simulink library "Backhoe_Lib"  (R2014a)
settings: Solver=ode45  StartTime=0.0  StopTime=10.0  RelTol=1e-3
undefined symbols (not defined in the file): cylinderGray, gcbh, pistonGray, rhoSteel, simmechanics, X, Y, Z
libraries: sm_lib x40, Backhoe_Lib x7, fl_lib x7, nesl_utility x2
(part 1 of 2)
Description:
  | Copyright 2008-2014 The MathWorks, Inc.
settings Model: Creator=MathWorks  LastModifiedBy=Olli

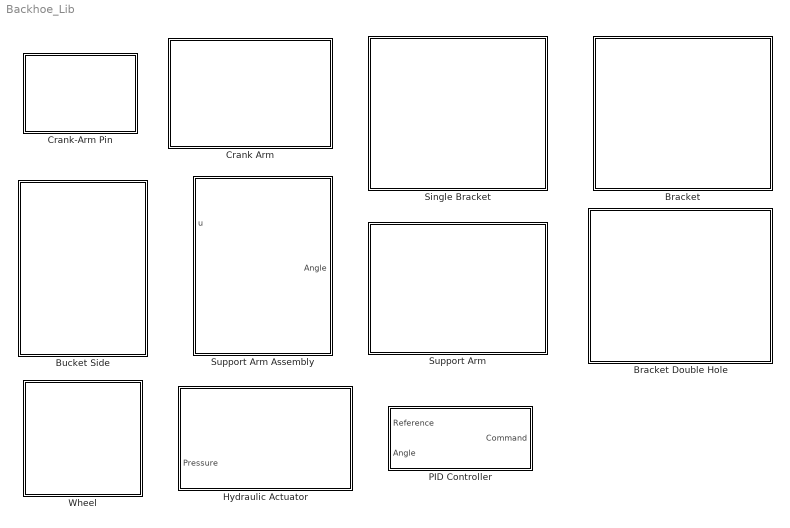
== system Backhoe_Lib ==
  Bracket : Subsystem  mask(Bracket){Hbracket=0.75, Wbracket=0.75, Tbracket=0.15, Dbracket=0.8, Hhole=0.5, Rhole=0.075, circlePoints=25, bracketColor=[0.8 0.8 0], rho=7780}
      mask prompts: Hbracket "Hbracket [m]"; Wbracket "Wbracket [m]"; Tbracket "Tbracket [m]"; Dbracket "Dbracket [m]"; Hhole "Hhole [m]"; Rhole "Rhole [m]"; circlePoints "Circle Mesh Resolution"; bracketColor "Bracket Color"; rho "Density [kg/m^3]"
      mask help:
      | Consists of the backhoe bracket assembly.
      |
      | Attachment points are:
      | B: The base of the bracket.
      | H: The center point between the two holes, which is configured for Revolute joints.
      |
      | Click on Help to view a schematic of the bracket, its configurable dimension parameters and attachment points (in red).
      mask init:
      | bracketPoints = [];
      | 
      | %% Bracket mold.
      | y = Hbracket - (Wbracket/2);
      | for i = 0:circlePoints
      |     angle = (i/circlePoints)*pi;
      |     bracketPoints = [bracketPoints; ...
      |                     (Wbracket/2)*cos(angle) (y+(Wbracket/2)*sin(angle))];
      | end
      | bracketPoints = [bracketPoints; ...
      |                  -Wbracket/2 0;0 0];
      |              
      | %% Hole
      | for i = 0:circlePoints*2
      |     angle = -pi/2 - (i/circlePoints)*pi;
      |     bracketPoints = [bracketPoints; ...
      |                     Rhole*cos(angle) (Hhole+(Rhole*sin(angle)))];
      | end
      | bracketPoints = [bracketPoints; ...
      |                  0 0;Wbracket/2 0];
      |                  
      | %% Uncomment to plot the cross-sections
      | % close all;
      | % figure;
      | % plot(bracketPoints(:,1),bracketPoints(:,2),'b*-');
      mask Help: web('Backhoe_Bracket.html');
      mask Display:
      | image(imread('Backhoe_Bracket_IMAGE.png'));
      | port_label('lconn',1,'B');
      | port_label('rconn',1,'H');
  Bracket Double Hole : Subsystem  mask(Bracket Double Hole){Hbracket=1, Wbracket=2, Tbracket=0.15, Dbracket=0.8, Hhole=0.5, Dhole=1.5, Rhole=0.1, Rfillet=0.4, Nc=25, bracketColor=[0.8 0.8 0], rho=7780}
      mask prompts: Hbracket "Hbracket [m]"; Wbracket "Wbracket [m]"; Tbracket "Tbracket [m]"; Dbracket "Dbracket [m]"; Hhole "Hhole [m]"; Dhole "Dhole [m]"; Rhole "Rhole [m]"; Rfillet "Rfillet [m]"; Nc "Circle Resolution (pts/rev)"; bracketColor "Bracket Color"; rho "Density [kg/m^3]"
      mask help:
      | Consists of the backhoe double-hole bracket assembly.
      |
      | Attachment points are:
      | B: The base of the bracket.
      | HL: The center point between the two left holes, which is configured for Revolute joints.
      | HR: The center point between the two right holes, which is configured for Revolute joints.
      |
      | Click on Help to view a schematic of the bracket, its configurable dimension parameters and attachment points (in red).
      mask init:
      | %% Right Hole
      | bracketPoints = [0 0; Dhole/2 0];
      | angle = linspace(-pi/2,-5*pi/2,Nc)';
      | bracketPoints = [bracketPoints; ...
      |                  (Dhole/2+Rhole*cos(angle)) (Hhole+Rhole*sin(angle))];
      | bracketPoints = [bracketPoints; Dhole/2 0];                 
      | 
      | %% Bracket Outer Boundary
      | bracketPoints = [bracketPoints; Wbracket/2 0];
      | x = Wbracket/2 - Rfillet;
      | y = Hbracket - Rfillet;
      | angle = linspace(0,pi/2,Nc/4)';
      | bracketPoints = [bracketPoints; ...
      |                  (x+Rfillet*cos(angle)) (y+Rfillet*sin(angle))];
      | 
      | angle = linspace(pi/2,pi,Nc/4)';             
      | bracketPoints = [bracketPoints; ...
      |                  (-x+Rfillet*cos(angle)) (y+Rfillet*sin(angle))];
      | bracketPoints = [bracketPoints; -Wbracket/2 0];
      |                  
      | %% Left Hole
      | bracketPoints = [bracketPoints;-Dhole/2 0];
      | angle = linspace(-pi/2,-5*pi/2,Nc)';
      | bracketPoints = [bracketPoints; ...
      |                  (-Dhole/2+Rhole*cos(angle)) (Hhole+Rhole*sin(angle))];
      | bracketPoints = [bracketPoints;-Dhole/2 0];
      mask Help: web('Backhoe_Bracket2.html');
      mask Display:
      | image(imread('Backhoe_Bracket2_IMAGE.png'));
      | port_label('lconn',1,'B');
      | port_label('rconn',1,'HR');
      | port_label('rconn',2,'HL');
  Bucket Side : Subsystem  mask(Bucket Side){bucketUpper=1.3, bucketLower=2, bucketHeight=2, bucketThickness=0.05, chordAngle=pi/6, Nc=45, color=[0.8 0.8 0], rho=7780}
      mask prompts: bucketUpper "Wupper [m]"; bucketLower "Wlower [m]"; bucketHeight "Hbucket [m]"; bucketThickness "Tbucket [m]"; chordAngle "alpha [radians]"; Nc "Circle Resolution (pts/rev)"; rho "Density [kg/m^3]"
      mask help:
      | Consists of the backhoe bucket side plate, which is used as an auxiliary library block inside the Bucket block.
      |
      | Click on Help to view a schematic of the bucket, its configurable dimension parameters and attachment points (in red).
      mask init:
      | bucketRadius = bucketHeight/(2*cos(chordAngle));
      | 
      | Nch = Nc*(pi-2*chordAngle)/(2*pi);
      | angle = linspace(-pi/2+chordAngle, pi/2-chordAngle,Nch)'; 
      | bucketSide = [(bucketRadius*cos(angle)-bucketRadius*sin(chordAngle)) ...
      |        bucketRadius*sin(angle)];
      | 
      | bucketSide = [ bucketSide; ...
      |               -bucketUpper bucketHeight/2; ...
      |               -bucketLower -(bucketHeight/2 - bucketThickness);...
      |               -bucketLower -bucketHeight/2];
      mask Help: web('Backhoe_Bucket.html');
      mask Display:
      | image(imread('Backhoe_Bucketside_IMAGE.png'));
      | port_label('rconn',1,'B');
  Crank Arm : Subsystem  mask(Crank Arm){L=1, W=0.25, T=0.1, D=0.75, R=0.05, Nc=25, color=[0.8 0.8 0], rho=7780}
      mask prompts: L "L [m]"; W "W [m]"; T "T [m]"; D "D [m]"; R "Rhole [m]"; Nc "Circle Resolution (pts/rev)"; rho "Density [kg/m^3]"
      mask help:
      | Parameterized bar with rounded ends and two holes for attachment.
      |
      | Attachment points are the left (L) and right (R) holes of the crank arm, which are configured for Revolute Joints.
      |
      | Click on Help to view a schematic of the bracket, its configurable dimension parameters and attachment points (in red).
      mask init:
      | crankPoints = [];
      | 
      | % Crank 1
      | x = (L - W)/2;
      | angle = linspace(-pi/2,pi/2,Nc/2)';
      | crankPoints = [crankPoints; ...
      |       (x + W*cos(angle)/2) W*sin(angle)/2];
      |   
      | x = D/2;
      | angle = linspace(pi/2,-3*pi/2,Nc)';
      | crankPoints = [crankPoints; ...
      |       (x + R*cos(angle)) R*sin(angle)];
      | 
      | crankPoints = [crankPoints;x W/2];
      | x = -D/2;
      | crankPoints = [crankPoints;x W/2];
      | 
      | angle = linspace(pi/2,-3*pi/2,Nc)';
      | crankPoints = [crankPoints; ...
      |       (x + R*cos(angle)) R*sin(angle)];
      | 
      | x = -(L - W)/2;
      | angle = linspace(pi/2,3*pi/2,Nc/2)';
      | crankPoints = [crankPoints; ...
      |       (x + W*cos(angle)/2) W*sin(angle)/2];
      mask Help: web('Backhoe_Crankarm.html');
      mask Display:
      | image(imread('Backhoe_Crankarm_IMAGE.png'));
      | port_label('lconn',1,'L');
      | port_label('rconn',1,'R');
  Crank-Arm Pin : Subsystem  mask(Crank Pin){R=0.1, L=1, T=0.1, color=[0.3 0.3 0.3], rho=7780}
      mask prompts: R "Radius [m]"; L "Length [m]"; T "Crank Arm Thickness [m]"; rho "Density [kg/m^3]"
      mask help:
      | Parameterized block for the two pins that extrude from the Upper Arm. These pins connect to the crank arms, which create a four-bar linkage with the Upper Arm and the Bucket.
      |
      | Attachment points are:
      | B: Base of the pin.
      | C: Crank arm attachment point which is configured for Revolute joints.
      mask Display:
      | image(repmat(imread('Backhoe_Crankpin_IMAGE.png'),[1 1 3]));
      | port_label('lconn',1,'C');
      | port_label('rconn',1,'B');
  Hydraulic Actuator : Subsystem  mask(Hydraulic Actuator){Lcyl=2.5, Rcyl=0.2, Lpist=2.5, Rpist=0.1, Lbase=0.65, Wbase=0.35, Rbp=0.075, Lbp=0.8, Whead=0.35, Lhead=0.65, Rhp=0.075, Lhp=0.9, circlePoints=25, cylColor=[0.6 0.6 0.6], rhoCyl=7780, pistColor=[0.4 0.4 0.4], rhoPist=7780, connColor=[0.3 0.3 0.3], rhoConn=7780}
      mask prompts: Lcyl "Lcyl [m]"; Rcyl "Rcyl [m]"; Lpist "Lpist [m]"; Rpist "Rpist [m]"; Lbase "Lbase [m]"; Wbase "Wbase [m]"; Rbp "Rbp [m]"; Lbp "Lbp [m]"; Whead "Whead [m]"; Lhead "Lhead [m]"; Rhp "Rhp [m]"; Lhp "Lhp [m]"; circlePoints "Circle Mesh Resolution"; cylColor "Cylinder Color"; rhoCyl "Cylinder Density [kg/m^3]"; pistColor "Piston Color"; rhoPist "Piston Density [kg/m^3]"; connColor "Connector Color"; rhoConn "Connector Density [kg/m^3]"
      mask help:
      | Consists of the backhoe hydraulic actuator assembly.
      |
      | Zero piston displacement corresponds to the piston and cylinder centers of mass in the same position. Positive piston displacement is outward motion, and negative piston displacement is inward motion.
      |
      | Attachment points are:
      | C: Center of the Cylinder base bracket hole.
      | H: Center of the Piston Head bracket hole.
      | Both attachment points are configured for Revolute joints.
      |
      | The Simulink Signal input port supplies a Pressure value P (in Pa) to a Simscape hydraulic network.
      |
      | Click on Help to view a schematic of the hydraulic actuator, its configurable dimension parameters and attachment points (in red).
      mask init:
      | % Hollow Cylinder cross-section
      | cylSection = [];
      | 
      | for i = 0:2*circlePoints
      |     angle = (i/circlePoints)*pi;
      |     cylSection = [cylSection; Rcyl*cos(angle) Rcyl*sin(angle)];
      | end
      | 
      | for i = 0:2*circlePoints
      |     angle = -(i/circlePoints)*pi;
      |     cylSection = [cylSection; Rpist*cos(angle) Rpist*sin(angle)];
      | end
      mask Help: web('Backhoe_Actuator.html');
      mask Display:
      | image(repmat(imread('Backhoe_Actuator_IMAGE.png'),[1 1 3]));
      | port_label('rconn',1,'H');
      | port_label('lconn',1,'C');
      | port_label('input',1,'P');
  PID Controller : Subsystem  mask(PID Controller){upperLim=inf, lowerLim=-inf, Kp=0, Ki=0, Kd=0, N=0}
      mask prompts: upperLim "Upper Limit [deg]"; lowerLim "Lower Limit [deg]"
      mask help: This block takes in a reference angle and measured angle, and uses a PID Controller with saturation to give a control command.
  Single Bracket : Subsystem  mask(Single Bracket){Hbracket=0.75, Wbracket=0.75, Tbracket=0.15, Hhole=0.5, Rhole=0.075, Nc=25, bracketColor=[0.8 0.8 0], rho=7780}
      mask prompts: Hbracket "Hbracket [m]"; Wbracket "Wbracket [m]"; Tbracket "Tbracket [m]"; Hhole "Hhole [m]"; Rhole "Rhole [m]"; Nc "Circle Resolution (pts/rev)"; bracketColor "Bracket Color"; rho "Density [kg/m^3]"
      mask help:
      | Consists of the backhoe single bracket assembly.
      |
      | Attachment points are:
      | B: The base of the bracket.
      | H: The center point of the hole, which is configured for Revolute joints.
      |
      | Click on Help to view a schematic of the bracket, its configurable dimension parameters and attachment points (in red).
      mask init:
      | bracketPoints = [];
      | 
      | %% Bracket mold.
      | y = Hbracket - (Wbracket/2);
      | angle = linspace(0,pi,Nc/2)';
      | bracketPoints = [(Wbracket/2)*cos(angle) (y+(Wbracket/2)*sin(angle))];
      | bracketPoints = [bracketPoints; ...
      |                  -Wbracket/2 0;0 0];
      |              
      | %% Hole
      | angle = linspace(3*pi/2,-pi/2,Nc)';
      | bracketPoints = [bracketPoints; ...
      |                  Rhole*cos(angle) (Hhole+(Rhole*sin(angle)))];
      | bracketPoints = [bracketPoints; ...
      |                  0 0;Wbracket/2 0];
      mask Help: web('Backhoe_Singlebracket.html');
      mask Display:
      | image(imread('Backhoe_Bracket1_IMAGE.png'));
      | port_label('lconn',1,'B');
      | port_label('rconn',1,'H');
  Support Arm : Subsystem  mask(Support Arm){Larm=2.5, Warm=0.5, Tarm=0.35, Dhole=2, Rhole=0.075, initAngle=45, Lfoot=2, Wfoot=1, Tfoot=0.2, Dconn=1, Hhole=0.3, Rfillet=0.4, Lpin=0.8, circlePoints=25, armColor=[0.8 0.8 0], bracketColor=[0.8 0.65 0], footColor=[0.8 0.8 0], pinColor=[0.3 0.3 0.3], rho=7780}
      mask prompts: Larm "Larm [m]"; Warm "Warm [m]"; Tarm "Tarm [m]"; Dhole "Dhole [m]"; Rhole "Rhole [m]"; initAngle "Initial Arm-Foot Angle [deg]"; Lfoot "Lfoot [m]"; Wfoot "Wfoot [m]"; Tfoot "Tfoot [m]"; Dconn "Dconn [m]"; Hhole "Hhole [m]"; Rfillet "Rfillet [m]"; Lpin "Lpin [m]"; circlePoints "Circle Mesh Resolution"; armColor "Arm Color"; bracketColor "Bracket Color"; footColor "Foot Color"; pinColor "Pin Color"; rho "Density [kg/m^3]"
      mask help:
      | Consists of the backhoe support arm that connects an arm, a bracket and a foot.
      |
      | Attachment points are:
      | SB: The free hole of the crank arm, which connects to the Shoulder Bracket.
      | PH: The free pin of the foot bracket, which connect to the piston head of a hydraulic actuator.
      | Both attachment points are configured for Revolute Joints.
      |
      | Click on Help to view a schematic of the support arm, its configurable dimension parameters and attachment points (in red).
      mask init:
      | armPoints = [];
      | x = (Larm - Warm)/2;
      | for i=0:circlePoints
      |    angle = -pi/2 + (i/circlePoints)*pi;
      |    armPoints = [armPoints; ...
      |       (x + Warm*cos(angle)/2) Warm*sin(angle)/2];
      | end
      | x = Dhole/2;
      | for i=0:circlePoints*2
      |    angle = pi/2 - (i/circlePoints)*pi;
      |    armPoints = [armPoints; ...
      |       (x + Rhole*cos(angle)) Rhole*sin(angle)];   
      | end
      | armPoints = [armPoints;x Warm/2];
      | x = -Dhole/2;
      | armPoints = [armPoints;x Warm/2];
      | for i=0:circlePoints*2
      |    angle = pi/2 - (i/circlePoints)*pi;
      |    armPoints = [armPoints; ...
      |       (x + Rhole*cos(angle)) Rhole*sin(angle)];   
      | end
      | x = -(Larm - Warm)/2;
      | for i=0:circlePoints
      |    angle = pi/2 + (i/circlePoints)*pi;
      |    armPoints = [armPoints; ...
      |       (x + Warm*cos(angle)/2) Warm*sin(angle)/2];
      | end
      mask Help: web('Backhoe_Supportarm.html');
      mask Display:
      | image(imread('Backhoe_Supportarm_IMAGE.png'));
      | port_label('lconn',1,'PH');
      | port_label('rconn',1,'SB');
  Support Arm Assembly : Subsystem  mask(Support Arm Assembly){Hbracket=0.8, Wbracket=1.75, Tbracket=0.15, Dbracket=0.8, HShoulderHole=0.5, DShoulderHole=1, RShoulderHole=0.075, RShoulderFillet=0.4, Larm=2.5, Warm=0.5, Tarm=0.35, Dhole=2, Rhole=0.075, AFAngle=45, Lpin=0.85, Lfoot=2, Wfoot=1, Tfoot=0.2, Dconn=1, Hhole=0.3, Rfillet=0.4, circlePoints=25, shoulderColor=[1 0.6 0], armColor=[1 0.8 0], bracketColor=[1 0.6 0], footColor=[1 0.8 0], pinColor=[0.5 0.5 0.5], pistonGray=pistonGray, cylinderGray=cylinderGray, rho=rhoSteel}
      mask prompts: Hbracket "Hbracket [m]"; Wbracket "Wbracket [m]"; Tbracket "Tbracket [m]"; Dbracket "Dbracket [m]"; HShoulderHole "HShoulderHole [m]"; DShoulderHole "DShoulderHole [m]"; RShoulderHole "RShoulderHole [m]"; RShoulderFillet "RShoulderFillet [m]"; Larm "Larm [m]"; Warm "Warm [m]"; Tarm "Tarm [m]"; Dhole "Dhole [m]"; Rhole "Rhole [m]"; AFAngle "Arm-Foot Angle [deg]"; Lpin "Lpin [m]"; Lfoot "Lfoot [m]"; Wfoot "Wfoot [m]"; Tfoot "Tfoot [m]"; Dconn "Dconn [m]"; Hhole "Hhole [m]"; Rfillet "Rfillet [m]"; circlePoints "Circle Mesh Resolution"; shoulderColor "Shoulder Bracket Color"; armColor "Arm Color"; bracketColor "Foot Bracket Color"; footColor "Foot Color"; pinColor "Pin Color"; pistonGray "Piston Color"; cylinderGray "Cylinder Color"; rho "Density [kg/m^3]"
      mask help:
      | Consists of a backhoe support arm, a shoulder bracket and a hydraulic actuator.
      |
      | Attachment points are:
      | MB: The base of the shoulder bracket, which connects rigidly to the Mounting Base.
      |
      | Inputs and outputs are:
      | u: The pressure to the hydraulic actuator.
      | a: The angle of the support arm, for sensing.
      |
      | Click on Help to view a schematic of the support arm assembly, its configurable dimension parameters and attachment points (in red).
      mask Help: web('Backhoe_Supportassembly.html');
      mask Display:
      | image(imread('Backhoe_Supportassembly_IMAGE.png'));
      | port_label('input',1,'u');
      | port_label('output',1,'a');
      | port_label('lconn',1,'MB');
  Wheel : Subsystem  mask(Wheel){Rwheel=0.5, Rtire=1, Raxle=0.075, W=0.75, circlePoints=30, tireColor=[0.1 0.1 0.1], rhoTire=1500, wheelColor=[0.6 0.6 0.6], rhoWheel=7780}
      mask prompts: Rwheel "Rwheel [m]"; Rtire "Rtire [m]"; Raxle "Raxle [m]"; W "Width [m]"; circlePoints "Circle Point Resolution"; tireColor "Tire Color"; rhoTire "Tire Density [kg/m^3]"; wheelColor "Wheel Color"; rhoWheel "Wheel Density [kg/m^3]"
      mask help:
      | Consists of the backhoe wheel assembly.
      |
      | Attachment points are:
      | A: The center of the wheel's axle.
      mask init:
      | % Wheel
      | wheelPoints = [];
      | for i = 0:circlePoints
      |    angle = pi*i/circlePoints;
      |    wheelPoints = [wheelPoints ; ...
      |                   Rwheel*cos(angle) Rwheel*sin(angle)];
      | end
      | for i = 0:2*circlePoints
      |    angle = pi - pi*i/circlePoints;
      |    wheelPoints = [wheelPoints ; ...
      |                   Raxle*cos(angle) Raxle*sin(angle)];
      | end
      | for i = 0:circlePoints
      |    angle = pi + pi*i/circlePoints;
      |    wheelPoints = [wheelPoints ; ...
      |                   Rwheel*cos(angle) Rwheel*sin(angle)];
      | end
      | 
      | % Tire
      | tirePoints = [];
      | for i = 0:circlePoints
      |    angle = pi*i/circlePoints;
      |    tirePoints = [tirePoints ; ...
      |                   Rtire*cos(angle) Rtire*sin(angle)];
      | end
      | for i = 0:2*circlePoints
      |    angle = pi - pi*i/circlePoints;
      |    tirePoints = [tirePoints ; ...
      |                   Rwheel*cos(angle) Rwheel*sin(angle)];
      | end
      | for i = 0:circlePoints
      |    angle = pi + pi*i/circlePoints;
      |    tirePoints = [tirePoints ; ...
      |                   Rtire*cos(angle) Rtire*sin(angle)];
      | end
      | 
      | % Rim
      | H = W*0.15;
      | k = H/(Rwheel^2);
      | vec = linspace(Rwheel,Raxle,10)';
      | rimPoints = [Raxle 0; vec  H-k*vec.^2];
      mask Display:
      | image(repmat(imread('Backhoe_Wheel_IMAGE.png'),[1 1 3]));
      | port_label('lconn',1,'A');

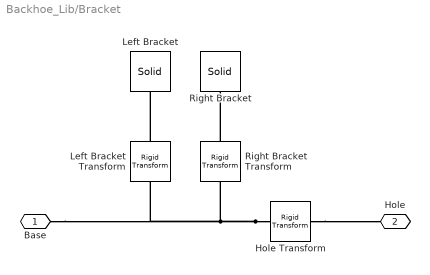
== system Backhoe_Lib/Bracket ==
  Hole Transform : sm_lib/Frames and Transforms/Rigid Transform  TranslationMethod=StandardAxis  TranslationLengthUnit=m  TranslationStandardAxis=+Z  TranslationStandardOffset=Hhole  TranslationCartesianOffset=[0 (Dbracket-Tbracket)/2 Hbracket/2]  TranslationROffset=0  TranslationROffsetUnits=m  TranslationZOffset=0  TranslationZOffsetUnits=m  TranslationThetaOffset=0  TranslationThetaOffsetUnits=deg  RotationMethod=AlignedAxes  RotationAngleUnits=deg  RotationStandardAxis=+X  RotationAngle=90  RotationArbitraryAxis=[0 0 1]  FollAlignAxisA=+X  BaseAlignAxisA=+X  FollAlignAxisB=+Y  BaseAlignAxisB=+Z  BlockFunction=simmechanics.library.frames_transforms.rigid_transform
  Left Bracket : sm_lib/Body Elements/Solid  InertiaType=CalculateFromGeometry  Mass=1  MassUnits=kg  CenterOfMass=[0 0 0]  CenterOfMassUnits=m  MomentsOfInertia=[1 1 1]  MomentsOfInertiaUnits=kg*m^2  ProductsOfInertia=[0 0 0]  ProductsOfInertiaUnits=kg*m^2  DensityBased=on  Density=rho  DensityUnits=kg/(m^3)  GraphicType=FromGeometry  MarkerShape=Sphere  MarkerSize=10  MarkerSizeUnits=m  GraphicVisPropType=SimpleVisualProperties  GraphicDiffuseColor=bracketColor  GraphicSpecularColor=[0.5 0.5 0.5 1.0]  GraphicAmbientColor=[0.15 0.15 0.15 1.0]  GraphicEmissiveColor=[0.0 0.0 0.0 1.0]  GraphicShininess=75  GraphicOpacity=1.0  GeometryShape=GeneralExtrusion  RectangleSize=[1 1]  RectangleSizeUnits=m  BrickDimensions=[Wbracket Tbracket Hbracket ]  BrickDimensionUnits=m  CylinderRadius=1  CylinderRadiusUnits=m  CylinderLength=1  CylinderLengthUnits=m  SphereRadius=1  SphereRadiusUnits=m  EllipsoidRadii=[1 1 1]  EllipsoidRadiiUnits=m  ExtrusionCrossSection=bracketPoints  ExtrusionCrossSectionUnits=m  ExtrusionLength=Tbracket  ExtrusionLengthUnits=m  PolygonNumSides=3  PolygonOuterRadius=1  PolygonOuterRadiusUnits=m  ExtGeomFileUnits=m  RevolutionCrossSection=[1 1; 1 -1; 2 -1; 2 1]  RevolutionCrossSectionUnits=m  RevolutionExtent=Full  RevolutionAngle=180  RevolutionAngleUnits=deg  BlockFunction=simmechanics.library.body_elements.solid
  Left Bracket Transform : sm_lib/Frames and Transforms/Rigid Transform  TranslationMethod=StandardAxis  TranslationLengthUnit=m  TranslationStandardAxis=-Y  TranslationStandardOffset=(Dbracket-Tbracket)/2  TranslationCartesianOffset=[0 0 0]  TranslationROffset=0  TranslationROffsetUnits=m  TranslationZOffset=0  TranslationZOffsetUnits=m  TranslationThetaOffset=0  TranslationThetaOffsetUnits=deg  RotationMethod=AlignedAxes  RotationAngleUnits=deg  RotationStandardAxis=+X  RotationAngle=90  RotationArbitraryAxis=[0 0 1]  FollAlignAxisA=+X  BaseAlignAxisA=+X  FollAlignAxisB=+Y  BaseAlignAxisB=+Z  BlockFunction=simmechanics.library.frames_transforms.rigid_transform
  Right Bracket : sm_lib/Body Elements/Solid  InertiaType=CalculateFromGeometry  Mass=1  MassUnits=kg  CenterOfMass=[0 0 0]  CenterOfMassUnits=m  MomentsOfInertia=[1 1 1]  MomentsOfInertiaUnits=kg*m^2  ProductsOfInertia=[0 0 0]  ProductsOfInertiaUnits=kg*m^2  DensityBased=on  Density=rho  DensityUnits=kg/(m^3)  GraphicType=FromGeometry  MarkerShape=Sphere  MarkerSize=10  MarkerSizeUnits=m  GraphicVisPropType=SimpleVisualProperties  GraphicDiffuseColor=bracketColor  GraphicSpecularColor=[0.5 0.5 0.5 1.0]  GraphicAmbientColor=[0.15 0.15 0.15 1.0]  GraphicEmissiveColor=[0.0 0.0 0.0 1.0]  GraphicShininess=75  GraphicOpacity=1.0  GeometryShape=GeneralExtrusion  RectangleSize=[1 1]  RectangleSizeUnits=m  BrickDimensions=[Wbracket Tbracket Hbracket ]  BrickDimensionUnits=m  CylinderRadius=1  CylinderRadiusUnits=m  CylinderLength=1  CylinderLengthUnits=m  SphereRadius=1  SphereRadiusUnits=m  EllipsoidRadii=[1 1 1]  EllipsoidRadiiUnits=m  ExtrusionCrossSection=bracketPoints  ExtrusionCrossSectionUnits=m  ExtrusionLength=Tbracket  ExtrusionLengthUnits=m  PolygonNumSides=3  PolygonOuterRadius=1  PolygonOuterRadiusUnits=m  ExtGeomFileUnits=m  RevolutionCrossSection=[1 1; 1 -1; 2 -1; 2 1]  RevolutionCrossSectionUnits=m  RevolutionExtent=Full  RevolutionAngle=180  RevolutionAngleUnits=deg  BlockFunction=simmechanics.library.body_elements.solid
  Right Bracket Transform : sm_lib/Frames and Transforms/Rigid Transform  TranslationMethod=StandardAxis  TranslationLengthUnit=m  TranslationStandardAxis=+Y  TranslationStandardOffset=(Dbracket-Tbracket)/2  TranslationCartesianOffset=[0 (Dbracket-Tbracket)/2 Hbracket/2]  TranslationROffset=0  TranslationROffsetUnits=m  TranslationZOffset=0  TranslationZOffsetUnits=m  TranslationThetaOffset=0  TranslationThetaOffsetUnits=deg  RotationMethod=AlignedAxes  RotationAngleUnits=deg  RotationStandardAxis=+X  RotationAngle=90  RotationArbitraryAxis=[0 0 1]  FollAlignAxisA=+X  BaseAlignAxisA=+X  FollAlignAxisB=+Y  BaseAlignAxisB=+Z  BlockFunction=simmechanics.library.frames_transforms.rigid_transform
  Base : PMIOPort  Port=1  Side=Left
  Hole : PMIOPort  Port=2  Side=Right
  connections:
  Hole Transform/LConn1 -- Base/RConn1 -- Left Bracket Transform/LConn1 -- Right Bracket Transform/LConn1
  Right Bracket Transform/RConn1 -- Right Bracket/RConn1
  Left Bracket Transform/RConn1 -- Left Bracket/RConn1
  Hole Transform/RConn1 -- Hole/RConn1

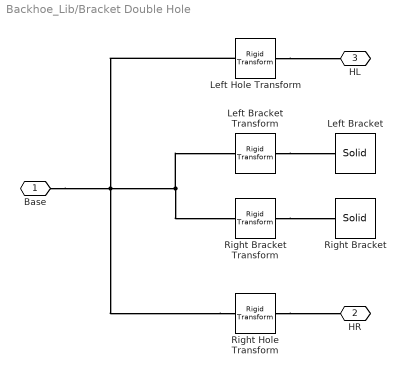
== system Backhoe_Lib/Bracket Double Hole ==
  Left Bracket : sm_lib/Body Elements/Solid  InertiaType=CalculateFromGeometry  Mass=1  MassUnits=kg  CenterOfMass=[0 0 0]  CenterOfMassUnits=m  MomentsOfInertia=[1 1 1]  MomentsOfInertiaUnits=kg*m^2  ProductsOfInertia=[0 0 0]  ProductsOfInertiaUnits=kg*m^2  DensityBased=on  Density=rho  DensityUnits=kg/(m^3)  GraphicType=FromGeometry  MarkerShape=Sphere  MarkerSize=10  MarkerSizeUnits=m  GraphicVisPropType=SimpleVisualProperties  GraphicDiffuseColor=bracketColor  GraphicSpecularColor=[0.5 0.5 0.5 1.0]  GraphicAmbientColor=[0.15 0.15 0.15 1.0]  GraphicEmissiveColor=[0.0 0.0 0.0 1.0]  GraphicShininess=75  GraphicOpacity=1.0  GeometryShape=GeneralExtrusion  RectangleSize=[1 1]  RectangleSizeUnits=m  BrickDimensions=[Wbracket Tbracket Hbracket ]  BrickDimensionUnits=m  CylinderRadius=1  CylinderRadiusUnits=m  CylinderLength=1  CylinderLengthUnits=m  SphereRadius=1  SphereRadiusUnits=m  EllipsoidRadii=[1 1 1]  EllipsoidRadiiUnits=m  ExtrusionCrossSection=bracketPoints  ExtrusionCrossSectionUnits=m  ExtrusionLength=Tbracket  ExtrusionLengthUnits=m  PolygonNumSides=3  PolygonOuterRadius=1  PolygonOuterRadiusUnits=m  ExtGeomFileUnits=m  RevolutionCrossSection=[1 1; 1 -1; 2 -1; 2 1]  RevolutionCrossSectionUnits=m  RevolutionExtent=Full  RevolutionAngle=180  RevolutionAngleUnits=deg  BlockFunction=simmechanics.library.body_elements.solid
  Left Bracket Transform : sm_lib/Frames and Transforms/Rigid Transform  TranslationMethod=StandardAxis  TranslationLengthUnit=m  TranslationStandardAxis=-Y  TranslationStandardOffset=(Dbracket-Tbracket)/2  TranslationCartesianOffset=[0 0 0]  TranslationROffset=0  TranslationROffsetUnits=m  TranslationZOffset=0  TranslationZOffsetUnits=m  TranslationThetaOffset=0  TranslationThetaOffsetUnits=deg  RotationMethod=AlignedAxes  RotationAngleUnits=deg  RotationStandardAxis=+X  RotationAngle=90  RotationArbitraryAxis=[0 0 1]  FollAlignAxisA=+X  BaseAlignAxisA=+X  FollAlignAxisB=+Y  BaseAlignAxisB=+Z  BlockFunction=simmechanics.library.frames_transforms.rigid_transform
  Left Hole Transform : sm_lib/Frames and Transforms/Rigid Transform  TranslationMethod=Cartesian  TranslationLengthUnit=m  TranslationStandardAxis=+Z  TranslationStandardOffset=0  TranslationCartesianOffset=[-Dhole/2 0 Hhole]  TranslationROffset=0  TranslationROffsetUnits=m  TranslationZOffset=0  TranslationZOffsetUnits=m  TranslationThetaOffset=0  TranslationThetaOffsetUnits=deg  RotationMethod=AlignedAxes  RotationAngleUnits=deg  RotationStandardAxis=+Z  RotationAngle=0  RotationArbitraryAxis=[0 0 1]  FollAlignAxisA=+X  BaseAlignAxisA=+X  FollAlignAxisB=+Y  BaseAlignAxisB=+Z  BlockFunction=simmechanics.library.frames_transforms.rigid_transform
  Right Bracket : sm_lib/Body Elements/Solid  InertiaType=CalculateFromGeometry  Mass=1  MassUnits=kg  CenterOfMass=[0 0 0]  CenterOfMassUnits=m  MomentsOfInertia=[1 1 1]  MomentsOfInertiaUnits=kg*m^2  ProductsOfInertia=[0 0 0]  ProductsOfInertiaUnits=kg*m^2  DensityBased=on  Density=rho  DensityUnits=kg/(m^3)  GraphicType=FromGeometry  MarkerShape=Sphere  MarkerSize=10  MarkerSizeUnits=m  GraphicVisPropType=SimpleVisualProperties  GraphicDiffuseColor=bracketColor  GraphicSpecularColor=[0.5 0.5 0.5 1.0]  GraphicAmbientColor=[0.15 0.15 0.15 1.0]  GraphicEmissiveColor=[0.0 0.0 0.0 1.0]  GraphicShininess=75  GraphicOpacity=1.0  GeometryShape=GeneralExtrusion  RectangleSize=[1 1]  RectangleSizeUnits=m  BrickDimensions=[Wbracket Tbracket Hbracket ]  BrickDimensionUnits=m  CylinderRadius=1  CylinderRadiusUnits=m  CylinderLength=1  CylinderLengthUnits=m  SphereRadius=1  SphereRadiusUnits=m  EllipsoidRadii=[1 1 1]  EllipsoidRadiiUnits=m  ExtrusionCrossSection=bracketPoints  ExtrusionCrossSectionUnits=m  ExtrusionLength=Tbracket  ExtrusionLengthUnits=m  PolygonNumSides=3  PolygonOuterRadius=1  PolygonOuterRadiusUnits=m  ExtGeomFileUnits=m  RevolutionCrossSection=[1 1; 1 -1; 2 -1; 2 1]  RevolutionCrossSectionUnits=m  RevolutionExtent=Full  RevolutionAngle=180  RevolutionAngleUnits=deg  BlockFunction=simmechanics.library.body_elements.solid
  Right Bracket Transform : sm_lib/Frames and Transforms/Rigid Transform  TranslationMethod=StandardAxis  TranslationLengthUnit=m  TranslationStandardAxis=+Y  TranslationStandardOffset=(Dbracket-Tbracket)/2  TranslationCartesianOffset=[0 (Dbracket-Tbracket)/2 Hbracket/2]  TranslationROffset=0  TranslationROffsetUnits=m  TranslationZOffset=0  TranslationZOffsetUnits=m  TranslationThetaOffset=0  TranslationThetaOffsetUnits=deg  RotationMethod=AlignedAxes  RotationAngleUnits=deg  RotationStandardAxis=+X  RotationAngle=90  RotationArbitraryAxis=[0 0 1]  FollAlignAxisA=+X  BaseAlignAxisA=+X  FollAlignAxisB=+Y  BaseAlignAxisB=+Z  BlockFunction=simmechanics.library.frames_transforms.rigid_transform
  Right Hole Transform : sm_lib/Frames and Transforms/Rigid Transform  TranslationMethod=Cartesian  TranslationLengthUnit=m  TranslationStandardAxis=+Z  TranslationStandardOffset=Hhole  TranslationCartesianOffset=[Dhole/2 0 Hhole]  TranslationROffset=0  TranslationROffsetUnits=m  TranslationZOffset=0  TranslationZOffsetUnits=m  TranslationThetaOffset=0  TranslationThetaOffsetUnits=deg  RotationMethod=AlignedAxes  RotationAngleUnits=deg  RotationStandardAxis=+X  RotationAngle=90  RotationArbitraryAxis=[0 0 1]  FollAlignAxisA=+X  BaseAlignAxisA=+X  FollAlignAxisB=+Y  BaseAlignAxisB=+Z  BlockFunction=simmechanics.library.frames_transforms.rigid_transform
  Base : PMIOPort  Port=1  Side=Left
  HR : PMIOPort  Port=2  Side=Right
  HL : PMIOPort  Port=3  Side=Right
  connections:
  Right Hole Transform/RConn1 -- HR/RConn1
  Right Bracket Transform/RConn1 -- Right Bracket/RConn1
  Right Hole Transform/LConn1 -- Left Hole Transform/LConn1 -- Base/RConn1 -- Left Bracket Transform/LConn1 -- Right Bracket Transform/LConn1
  Left Bracket Transform/RConn1 -- Left Bracket/RConn1
  Left Hole Transform/RConn1 -- HL/RConn1

== system Backhoe_Lib/Bucket Side ==
  Bucket Side : sm_lib/Body Elements/Solid  InertiaType=CalculateFromGeometry  Mass=1  MassUnits=kg  CenterOfMass=[0 0 0]  CenterOfMassUnits=m  MomentsOfInertia=[1 1 1]  MomentsOfInertiaUnits=kg*m^2  ProductsOfInertia=[0 0 0]  ProductsOfInertiaUnits=kg*m^2  DensityBased=on  Density=rho  DensityUnits=kg/(m^3)  GraphicType=FromGeometry  MarkerShape=Sphere  MarkerSize=10  MarkerSizeUnits=m  GraphicVisPropType=SimpleVisualProperties  GraphicDiffuseColor=bucketColor  GraphicSpecularColor=[0.5 0.5 0.5 1.0]  GraphicAmbientColor=[0.15 0.15 0.15 1.0]  GraphicEmissiveColor=[0.0 0.0 0.0 1.0]  GraphicShininess=75  GraphicOpacity=1.0  GeometryShape=GeneralExtrusion  RectangleSize=[1 1]  RectangleSizeUnits=m  BrickDimensions=[1 1 1]  BrickDimensionUnits=m  CylinderRadius=1  CylinderRadiusUnits=m  CylinderLength=1  CylinderLengthUnits=m  SphereRadius=1  SphereRadiusUnits=m  EllipsoidRadii=[1 1 1]  EllipsoidRadiiUnits=m  ExtrusionCrossSection=bucketSide  ExtrusionCrossSectionUnits=m  ExtrusionLength=bucketThickness  ExtrusionLengthUnits=m  PolygonNumSides=3  PolygonOuterRadius=1  PolygonOuterRadiusUnits=m  ExtGeomFileType=STL  ExtGeomFileUnits=m  RevolutionCrossSection=[1 1; 1 -1; 2 -1; 2 1]  RevolutionCrossSectionUnits=m  RevolutionExtent=Full  RevolutionAngle=180  RevolutionAngleUnits=deg  BlockFunction=simmechanics.library.body_elements.solid
  Bucket : PMIOPort  Port=1  Side=Right
  connections:
  Bucket Side/RConn1 -- Bucket/RConn1

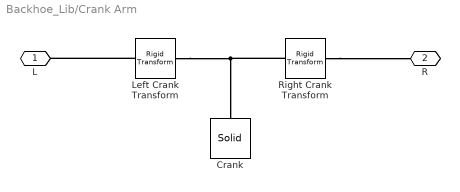
== system Backhoe_Lib/Crank Arm ==
  Crank : sm_lib/Body Elements/Solid  InertiaType=CalculateFromGeometry  Mass=1  MassUnits=kg  CenterOfMass=[0 0 0]  CenterOfMassUnits=m  MomentsOfInertia=[1 1 1]  MomentsOfInertiaUnits=kg*m^2  ProductsOfInertia=[0 0 0]  ProductsOfInertiaUnits=kg*m^2  DensityBased=on  Density=rho  DensityUnits=kg/(m^3)  GraphicType=FromGeometry  MarkerShape=Sphere  MarkerSize=10  MarkerSizeUnits=m  GraphicVisPropType=SimpleVisualProperties  GraphicDiffuseColor=color  GraphicSpecularColor=[0.5 0.5 0.5 1.0]  GraphicAmbientColor=[0.15 0.15 0.15 1.0]  GraphicEmissiveColor=[0.0 0.0 0.0 1.0]  GraphicShininess=75  GraphicOpacity=1.0  GeometryShape=GeneralExtrusion  RectangleSize=[1 1]  RectangleSizeUnits=m  BrickDimensions=[1 1 1]  BrickDimensionUnits=m  CylinderRadius=1  CylinderRadiusUnits=m  CylinderLength=1  CylinderLengthUnits=m  SphereRadius=1  SphereRadiusUnits=m  EllipsoidRadii=[1 1 1]  EllipsoidRadiiUnits=m  ExtrusionCrossSection=crankPoints  ExtrusionCrossSectionUnits=m  ExtrusionLength=T  ExtrusionLengthUnits=m  PolygonNumSides=3  PolygonOuterRadius=1  PolygonOuterRadiusUnits=m  ExtGeomFileUnits=m  RevolutionCrossSection=[1 1; 1 -1; 2 -1; 2 1]  RevolutionCrossSectionUnits=m  RevolutionExtent=Full  RevolutionAngle=180  RevolutionAngleUnits=deg  BlockFunction=simmechanics.library.body_elements.solid
  Left Crank Transform : sm_lib/Frames and Transforms/Rigid Transform  TranslationMethod=StandardAxis  TranslationLengthUnit=m  TranslationStandardAxis=-X  TranslationStandardOffset=D/2  TranslationCartesianOffset=[0 0 0]  TranslationROffset=0  TranslationROffsetUnits=m  TranslationZOffset=0  TranslationZOffsetUnits=m  TranslationThetaOffset=0  TranslationThetaOffsetUnits=deg  RotationMethod=None  RotationAngleUnits=deg  RotationStandardAxis=+Z  RotationAngle=0  RotationArbitraryAxis=[0 0 1]  FollAlignAxisA=+X  BaseAlignAxisA=+Y  FollAlignAxisB=+Y  BaseAlignAxisB=+Z  BlockFunction=simmechanics.library.frames_transforms.rigid_transform
  Right Crank Transform : sm_lib/Frames and Transforms/Rigid Transform  TranslationMethod=StandardAxis  TranslationLengthUnit=m  TranslationStandardAxis=+X  TranslationStandardOffset=D/2  TranslationCartesianOffset=[0 0 0]  TranslationROffset=0  TranslationROffsetUnits=m  TranslationZOffset=0  TranslationZOffsetUnits=m  TranslationThetaOffset=0  TranslationThetaOffsetUnits=deg  RotationMethod=None  RotationAngleUnits=deg  RotationStandardAxis=+Z  RotationAngle=0  RotationArbitraryAxis=[0 0 1]  FollAlignAxisA=+X  BaseAlignAxisA=+Y  FollAlignAxisB=+Y  BaseAlignAxisB=+Z  BlockFunction=simmechanics.library.frames_transforms.rigid_transform
  L : PMIOPort  Port=1  Side=Left
  R : PMIOPort  Port=2  Side=Right
  connections:
  Left Crank Transform/RConn1 -- L/RConn1
  Left Crank Transform/LConn1 -- Right Crank Transform/LConn1 -- Crank/RConn1
  Right Crank Transform/RConn1 -- R/RConn1

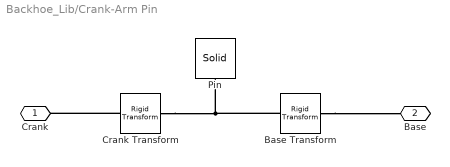
== system Backhoe_Lib/Crank-Arm Pin ==
  Base Transform : sm_lib/Frames and Transforms/Rigid Transform  TranslationMethod=StandardAxis  TranslationLengthUnit=m  TranslationStandardAxis=-Z  TranslationStandardOffset=L/2  TranslationCartesianOffset=[0 0 0]  TranslationROffset=0  TranslationROffsetUnits=m  TranslationZOffset=0  TranslationZOffsetUnits=m  TranslationThetaOffset=0  TranslationThetaOffsetUnits=deg  RotationMethod=None  RotationAngleUnits=deg  RotationStandardAxis=+Z  RotationAngle=0  RotationArbitraryAxis=[0 0 1]  FollAlignAxisA=+X  BaseAlignAxisA=+Y  FollAlignAxisB=+Y  BaseAlignAxisB=+Z  BlockFunction=simmechanics.library.frames_transforms.rigid_transform
  Crank Transform : sm_lib/Frames and Transforms/Rigid Transform  TranslationMethod=StandardAxis  TranslationLengthUnit=m  TranslationStandardAxis=+Z  TranslationStandardOffset=L/2 - 0.65*T  TranslationCartesianOffset=[0 0 0]  TranslationROffset=0  TranslationROffsetUnits=m  TranslationZOffset=0  TranslationZOffsetUnits=m  TranslationThetaOffset=0  TranslationThetaOffsetUnits=deg  RotationMethod=None  RotationAngleUnits=deg  RotationStandardAxis=+Z  RotationAngle=0  RotationArbitraryAxis=[0 0 1]  FollAlignAxisA=+X  BaseAlignAxisA=+Y  FollAlignAxisB=+Y  BaseAlignAxisB=+Z  BlockFunction=simmechanics.library.frames_transforms.rigid_transform
  Pin : sm_lib/Body Elements/Solid  InertiaType=CalculateFromGeometry  Mass=1  MassUnits=kg  CenterOfMass=[0 0 0]  CenterOfMassUnits=m  MomentsOfInertia=[1 1 1]  MomentsOfInertiaUnits=kg*m^2  ProductsOfInertia=[0 0 0]  ProductsOfInertiaUnits=kg*m^2  DensityBased=on  Density=rho  DensityUnits=kg/(m^3)  GraphicType=FromGeometry  MarkerShape=Sphere  MarkerSize=10  MarkerSizeUnits=m  GraphicVisPropType=SimpleVisualProperties  GraphicDiffuseColor=color  GraphicSpecularColor=[0.5 0.5 0.5 1.0]  GraphicAmbientColor=[0.15 0.15 0.15 1.0]  GraphicEmissiveColor=[0.0 0.0 0.0 1.0]  GraphicShininess=75  GraphicOpacity=1.0  GeometryShape=Cylinder  RectangleSize=[1 1]  RectangleSizeUnits=m  BrickDimensions=[1 1 1]  BrickDimensionUnits=m  CylinderRadius=R  CylinderRadiusUnits=m  CylinderLength=L  CylinderLengthUnits=m  SphereRadius=1  SphereRadiusUnits=m  EllipsoidRadii=[1 1 1]  EllipsoidRadiiUnits=m  ExtrusionCrossSection=[1 0]  ExtrusionCrossSectionUnits=m  ExtrusionLength=1  ExtrusionLengthUnits=m  PolygonNumSides=3  PolygonOuterRadius=1  PolygonOuterRadiusUnits=m  ExtGeomFileUnits=m  RevolutionCrossSection=[1 1; 1 -1; 2 -1; 2 1]  RevolutionCrossSectionUnits=m  RevolutionExtent=Full  RevolutionAngle=180  RevolutionAngleUnits=deg  BlockFunction=simmechanics.library.body_elements.solid
  Crank : PMIOPort  Port=1  Side=Left
  Base : PMIOPort  Port=2  Side=Right
  connections:
  Crank Transform/RConn1 -- Crank/RConn1
  Crank Transform/LConn1 -- Base Transform/LConn1 -- Pin/RConn1
  Base Transform/RConn1 -- Base/RConn1

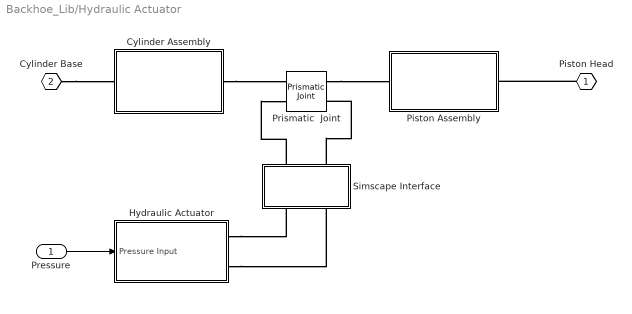
== system Backhoe_Lib/Hydraulic Actuator ==
  Pressure : Inport
  Cylinder Assembly : Subsystem
  Hydraulic Actuator : Subsystem
  Piston Assembly : Subsystem
  Prismatic  Joint : sm_lib/Joints/Prismatic Joint  SenseConstraintForce=off  SenseConstraintForceX=off  SenseConstraintForceY=off  SenseConstraintForceZ=off  SenseConstraintTorque=off  SenseConstraintTorqueX=off  SenseConstraintTorqueY=off  SenseConstraintTorqueZ=off  SenseTotalForce=off  SenseTotalForceX=off  SenseTotalForceY=off  SenseTotalForceZ=off  SenseTotalTorque=off  SenseTotalTorqueX=off  SenseTotalTorqueY=off  SenseTotalTorqueZ=off  CompositeWrenchDir=FollowerOnBase  CompositeWrenchFrame=BaseFrame  EquilibriumPosition=0  EquilibriumPositionUnits=m  SpringStiffness=0  SpringStiffnessUnits=N/m  DampingCoefficient=0  DampingCoefficientUnits=N/(m/s)  TorqueActuationMode=InputTorque  MotionActuationMode=ComputedMotion  SensePosition=off  SenseVelocity=on  SenseAcceleration=off  SenseTorqueForce=off  PositionTargetValue=0  PositionTargetValueUnits=m  PositionTargetSpecify=off  PositionTargetPriority=Low  VelocityTargetValue=0  VelocityTargetValueUnits=m/s  VelocityTargetSpecify=off  VelocityTargetPriority=High  BlockFunction=simmechanics.library.joints.prismatic_joint
  Simscape Interface : Subsystem
  Piston Head : PMIOPort  Port=1  Side=Right
  Cylinder Base : PMIOPort  Port=2  Side=Left
  wires:
  Pressure/1 -> Hydraulic Actuator/1(Pressure Input)
  connections:
  Cylinder Base/RConn1 -- Cylinder Assembly/RConn1
  Cylinder Assembly/LConn1 -- Prismatic  Joint/LConn1
  Prismatic  Joint/RConn1 -- Piston Assembly/LConn1
  Piston Head/RConn1 -- Piston Assembly/RConn1
  Hydraulic Actuator/RConn1 -- Simscape Interface/RConn1
  Simscape Interface/LConn2 -- Prismatic  Joint/RConn2
  Simscape Interface/LConn1 -- Prismatic  Joint/LConn2
  Hydraulic Actuator/RConn2 -- Simscape Interface/RConn2

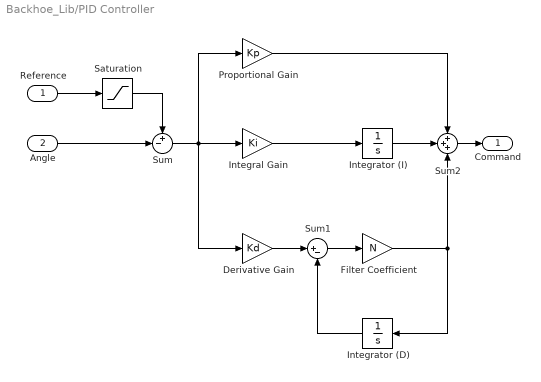
== system Backhoe_Lib/PID Controller ==
  Reference : Inport
  Angle : Inport  Port=2
  Derivative Gain : Gain  Gain=Kd
  Filter Coefficient : Gain  Gain=N
  Integral Gain : Gain  Gain=Ki
  Integrator (D) : Integrator
  Integrator (I) : Integrator
  Proportional Gain : Gain  Gain=Kp
  Saturation : Saturate  UpperLimit=upperLim  LowerLimit=lowerLim
  Sum : Sum  Inputs=+-|
  Sum1 : Sum  Inputs=|+-
  Sum2 : Sum  Inputs=+++
  Command : Outport
  wires:
  Saturation/1 -> Sum/1
  Angle/1 -> Sum/2
  Reference/1 -> Saturation/1
  Sum/1 -> Integral Gain/1, Proportional Gain/1, Derivative Gain/1
  Sum2/1 -> Command/1
  Integrator (I)/1 -> Sum2/2
  Integrator (D)/1 -> Sum1/2
  Filter Coefficient/1 -> Integrator (D)/1, Sum2/3
  Sum1/1 -> Filter Coefficient/1
  Derivative Gain/1 -> Sum1/1
  Integral Gain/1 -> Integrator (I)/1
  Proportional Gain/1 -> Sum2/1

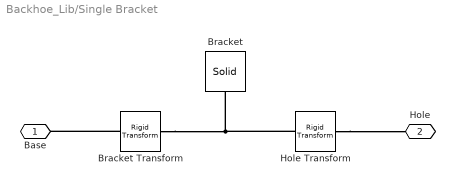
== system Backhoe_Lib/Single Bracket ==
  Bracket : sm_lib/Body Elements/Solid  InertiaType=CalculateFromGeometry  Mass=1  MassUnits=kg  CenterOfMass=[0 0 0]  CenterOfMassUnits=m  MomentsOfInertia=[1 1 1]  MomentsOfInertiaUnits=kg*m^2  ProductsOfInertia=[0 0 0]  ProductsOfInertiaUnits=kg*m^2  DensityBased=on  Density=rho  DensityUnits=kg/(m^3)  GraphicType=FromGeometry  MarkerShape=Sphere  MarkerSize=10  MarkerSizeUnits=m  GraphicVisPropType=SimpleVisualProperties  GraphicDiffuseColor=bracketColor  GraphicSpecularColor=[0.5 0.5 0.5 1.0]  GraphicAmbientColor=[0.15 0.15 0.15 1.0]  GraphicEmissiveColor=[0.0 0.0 0.0 1.0]  GraphicShininess=75  GraphicOpacity=1.0  GeometryShape=GeneralExtrusion  RectangleSize=[1 1]  RectangleSizeUnits=m  BrickDimensions=[Wbracket Tbracket Hbracket ]  BrickDimensionUnits=m  CylinderRadius=1  CylinderRadiusUnits=m  CylinderLength=1  CylinderLengthUnits=m  SphereRadius=1  SphereRadiusUnits=m  EllipsoidRadii=[1 1 1]  EllipsoidRadiiUnits=m  ExtrusionCrossSection=bracketPoints  ExtrusionCrossSectionUnits=m  ExtrusionLength=Tbracket  ExtrusionLengthUnits=m  PolygonNumSides=3  PolygonOuterRadius=1  PolygonOuterRadiusUnits=m  ExtGeomFileUnits=m  RevolutionCrossSection=[1 1; 1 -1; 2 -1; 2 1]  RevolutionCrossSectionUnits=m  RevolutionExtent=Full  RevolutionAngle=180  RevolutionAngleUnits=deg  BlockFunction=simmechanics.library.body_elements.solid
  Bracket Transform : sm_lib/Frames and Transforms/Rigid Transform  TranslationMethod=None  TranslationLengthUnit=m  TranslationStandardAxis=-Y  TranslationStandardOffset=0  TranslationCartesianOffset=[0 0 0]  TranslationROffset=0  TranslationROffsetUnits=m  TranslationZOffset=0  TranslationZOffsetUnits=m  TranslationThetaOffset=0  TranslationThetaOffsetUnits=deg  RotationMethod=AlignedAxes  RotationAngleUnits=deg  RotationStandardAxis=+X  RotationAngle=90  RotationArbitraryAxis=[0 0 1]  FollAlignAxisA=+X  BaseAlignAxisA=+X  FollAlignAxisB=+Y  BaseAlignAxisB=+Z  BlockFunction=simmechanics.library.frames_transforms.rigid_transform
  Hole Transform : sm_lib/Frames and Transforms/Rigid Transform  TranslationMethod=StandardAxis  TranslationLengthUnit=m  TranslationStandardAxis=+Y  TranslationStandardOffset=Hhole  TranslationCartesianOffset=[0 0 0]  TranslationROffset=0  TranslationROffsetUnits=m  TranslationZOffset=0  TranslationZOffsetUnits=m  TranslationThetaOffset=0  TranslationThetaOffsetUnits=deg  RotationMethod=None  RotationAngleUnits=deg  RotationStandardAxis=+X  RotationAngle=90  RotationArbitraryAxis=[0 0 1]  FollAlignAxisA=+X  BaseAlignAxisA=+X  FollAlignAxisB=+Y  BaseAlignAxisB=+Z  BlockFunction=simmechanics.library.frames_transforms.rigid_transform
  Base : PMIOPort  Port=1  Side=Left
  Hole : PMIOPort  Port=2  Side=Right
  connections:
  Hole Transform/LConn1 -- Bracket Transform/RConn1 -- Bracket/RConn1
  Hole Transform/RConn1 -- Hole/RConn1
  Bracket Transform/LConn1 -- Base/RConn1
